simulink model "cascaded_filter"  (Simulink 6.0)
settings: Solver=ode45  StartTime=0.0  StopTime=10.0  RelTol=1e-3
model workspace (MAT data in the model file):
  L = [4.47e-09 1.86e-06 8.93e-09]
  C = [1.007e-09 2.4e-12 5.04e-10]
undefined symbols (not defined in the file or in its folder): Fs, rfckt
libraries: rfports1 x6, rfblackbox1 x4, dspsnks4 x3, rftxlines1 x2, rfladderfilters1 x1, dspsrcs4 x1
settings Model: Creator=ashivapr  LastModifiedBy=rzeng  ProdHWDeviceType=Specified  UpdateModelReferenceTargets=IfOutOfDate
settings DataIOCC: SaveOutput=off  SaveTime=off  SignalLoggingName=logsOut
settings DebuggingCC: CheckExecutionContextPreStartOutputMsg=on  CheckExecutionContextRuntimeOutputMsg=on  SolverPrmCheckMsg=none
settings HardwareCC: ProdHWDeviceType=Specified
settings ModelReferenceCC: UpdateModelReferenceTargets=IfOutOfDate
settings GRTTargetCC: UtilityFuncGeneration=Automatic  LifeSpan=inf
settings SFSimCC: SFSimApplyToAllLibs=on  SFSimBuildMode=Incremental

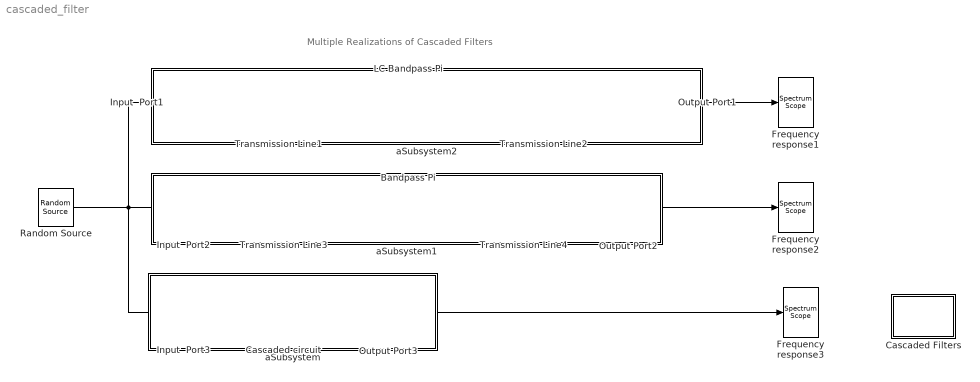
== system cascaded_filter ==
  note: Multiple Realizations of Cascaded Filters
  Bandpass Pi : rfblackbox1/General  Circuit Element  PhysicalDomain=rfsystemsdomain  SubClassName=general-circuit-element  LeftPortType=p1  RightPortType=p1  LConnTagsString=__newl0  RConnTagsString=__newr0  Ckt=rfckt.lcbandpasspi('L', L ,'C',C)  DisplayData=off  PlotFreq=Derived from Input Port parameters  PlotFreqNoSim=User specified  Freq=[70e6:1.0e5:80e6]  AllPlotType=X-Y plane  NetworkData=S21  SmithData=S11  PolarData=S11  ComplexFormat=Magnitude (decibels)  DBFormat=Magnitude (decibels)  NoneFormat=None
  Cascaded Filters : Subsystem  EnableExecutionContextPropagation=on
      mask Display: disp('Info')
  Cascaded circuit : rfblackbox1/General  Circuit Element  PhysicalDomain=rfsystemsdomain  SubClassName=general-circuit-element  LeftPortType=p1  RightPortType=p1  LConnTagsString=__newl0  RConnTagsString=__newr0  Ckt=rfckt.cascade('Ckts',{rfckt.txline,rfckt.lcbandpasspi('L', L, 'C',C), rfckt.txline})  DisplayData=off  PlotFreq=Derived from Input Port parameters  PlotFreqNoSim=User specified  Freq=[70e6:1.0e5:80e6]  AllPlotType=X-Y plane  NetworkData=S21  SmithData=S11  PolarData=S11  ComplexFormat=Magnitude (decibels)  DBFormat=Magnitude (decibels)  NoneFormat=None
  Frequency response1 : dspsnks4/Spectrum Scope  ScopeProperties=off  Domain=Frequency  HorizSpan=1  UseBuffer=off  BufferSize=128  Overlap=64  inpFftLenInherit=off  FFTlength=1024  numAvg=20  DisplayProperties=off  AxisGrid=on  Memory=off  FrameNumber=off  AxisLegend=off  AxisZoom=off  OpenScopeAtSimStart=on  OpenScopeImmediately=off  FigPos=[39 353 295 178]  AxisProperties=off  XUnits=Hertz  XRange=[-Fs/2...Fs/2]  InheritXIncr=on  XIncr=1.0  XLabel=Samples  YUnits=dB  YLabel=Magnitude, dB  LineProperties=on  LineColors=[0 0 1]
      settings: YMin=-21.8531881151715  YMax=-0.111894463142355
  Frequency response2 : dspsnks4/Spectrum Scope  ScopeProperties=off  Domain=Frequency  HorizSpan=1  UseBuffer=off  BufferSize=128  Overlap=64  inpFftLenInherit=off  FFTlength=1024  numAvg=20  DisplayProperties=off  AxisGrid=on  Memory=off  FrameNumber=off  AxisLegend=off  AxisZoom=off  OpenScopeAtSimStart=on  OpenScopeImmediately=off  FigPos=[342 353 294 178]  AxisProperties=off  XUnits=Hertz  XRange=[-Fs/2...Fs/2]  InheritXIncr=on  XIncr=1.0  XLabel=Samples  YUnits=dB  YLabel=Magnitude, dB  LineProperties=on  LineColors=[1 0 0]
      settings: YMin=-21.8644242577982  YMax=-0.721656811847852
  Frequency response3 : dspsnks4/Spectrum Scope  ScopeProperties=off  Domain=Frequency  HorizSpan=1  UseBuffer=off  BufferSize=128  Overlap=64  inpFftLenInherit=off  FFTlength=1024  numAvg=20  DisplayProperties=off  AxisGrid=on  Memory=off  FrameNumber=off  AxisLegend=off  AxisZoom=off  OpenScopeAtSimStart=on  OpenScopeImmediately=off  FigPos=[644 354 297 179]  AxisProperties=off  XUnits=Hertz  XRange=[-Fs/2...Fs/2]  InheritXIncr=on  XIncr=1.0  XLabel=Samples  YUnits=dB  YLabel=Magnitude, dB  LineProperties=on  LineColors=[0 0 0]
      settings: YMin=-21.7603958691771  YMax=-0.180062979467108
  Input  Port1 : rfports1/Input Port  Description=source block  MaxLength=128  Fc=75e6  Ts=1e-7  Zs=50  NoiseFlag=off  seed=67987  GoToTag=AAEGBHDRJLOGNSMOUDGJWHR
  Input  Port2 : rfports1/Input Port  Description=source block  MaxLength=128  Fc=75e6  Ts=1e-7  Zs=50  NoiseFlag=off  seed=67987  GoToTag=BBAACIESKMPHOTNPVEHKXIS
  Input  Port3 : rfports1/Input Port  Description=source block  MaxLength=128  Fc=75e6  Ts=1e-7  Zs=50  NoiseFlag=off  seed=67987  GoToTag=ACBBDJFALNQIAUOQWFILYJT
  LC Bandpass Pi : rfladderfilters1/LC Bandpass Pi  PhysicalDomain=rfsystemsdomain  SubClassName=lcbandpasspi  LeftPortType=p1  RightPortType=p1  LConnTagsString=__newl0  RConnTagsString=__newr0  L=L  C=C  DisplayData=off  PlotFreq=Derived from Input Port parameters  PlotFreqNoSim=User specified  Freq=[70e6:1.0e5:80e6]  AllPlotType=X-Y plane  NetworkData=S21  SmithData=S11  PolarData=S11  ComplexFormat=Magnitude (decibels)  DBFormat=Magnitude (decibels)  NoneFormat=None
  Output Port1 : rfports1/Output Port  Zl=100  num_Models=1  GoToTag=AAEGBHDRJLOGNSMOUDGJWHR  DisplayData=off  PlotFreq=Derived from Input Port parameters  Freq=1e9:1e8:3e9  AllPlotType=Composite data  NoBudgetPlot=Composite data  NetworkData=S11  SmithData=S11  PolarData=S11  ComplexFormat=Magnitude (decibels)  DBFormat=Magnitude (decibels)  DBMFormat=dBm  NoneFormat=None
  Output Port2 : rfports1/Output Port  Zl=100  num_Models=1  GoToTag=BBAACIESKMPHOTNPVEHKXIS  DisplayData=off  PlotFreq=Derived from Input Port parameters  Freq=1e9:1e8:3e9  AllPlotType=Composite data  NoBudgetPlot=Composite data  NetworkData=S11  SmithData=S11  PolarData=S11  ComplexFormat=Magnitude (decibels)  DBFormat=Magnitude (decibels)  DBMFormat=dBm  NoneFormat=None
  Output Port3 : rfports1/Output Port  Zl=100  num_Models=1  GoToTag=ACBBDJFALNQIAUOQWFILYJT  DisplayData=off  PlotFreq=Derived from Input Port parameters  Freq=1e9:1e8:3e9  AllPlotType=Composite data  NoBudgetPlot=Composite data  NetworkData=S11  SmithData=S11  PolarData=S11  ComplexFormat=Magnitude (decibels)  DBFormat=Magnitude (decibels)  DBMFormat=dBm  NoneFormat=None
  Random Source : dspsrcs4/Random Source  SrcType=Gaussian  NormMethod=Ziggurat  CltLength=12  Min=0  Max=1  Mean=0  Var=1  RepMode=Not repeatable  Seed=1  Inherit=off  SampMode=Discrete  SampTime=1e-7  SampFrame=256  DataType=Double  OutComplex=Complex
  Transmission Line1 : rftxlines1/Transmission Line  PhysicalDomain=rfsystemsdomain  SubClassName=txline  LeftPortType=p1  RightPortType=p1  LConnTagsString=__newl0  RConnTagsString=__newr0  Z0=50  PV=299792458  Loss=0  LineLength=0.01  StubMode=Not a stub  Termination=Open  DisplayData=off  PlotFreq=Derived from Input Port parameters  PlotFreqNoSim=User specified  Freq=[70e6:1.0e5:80e6]  AllPlotType=X-Y plane  NetworkData=S21  SmithData=S11  PolarData=S11  ComplexFormat=Magnitude (decibels)  DBFormat=Magnitude (decibels)  NoneFormat=None
  Transmission Line2 : rftxlines1/Transmission Line  PhysicalDomain=rfsystemsdomain  SubClassName=txline  LeftPortType=p1  RightPortType=p1  LConnTagsString=__newl0  RConnTagsString=__newr0  Z0=50  PV=299792458  Loss=0  LineLength=0.01  StubMode=Not a stub  Termination=Open  DisplayData=off  PlotFreq=Derived from Input Port parameters  PlotFreqNoSim=User specified  Freq=[70e6:1.0e5:80e6]  AllPlotType=X-Y plane  NetworkData=S21  SmithData=S11  PolarData=S11  ComplexFormat=Magnitude (decibels)  DBFormat=Magnitude (decibels)  NoneFormat=None
  Transmission Line3 : rfblackbox1/General  Circuit Element  PhysicalDomain=rfsystemsdomain  SubClassName=general-circuit-element  LeftPortType=p1  RightPortType=p1  LConnTagsString=__newl0  RConnTagsString=__newr0  Ckt=rfckt.txline  DisplayData=off  PlotFreq=Derived from Input Port parameters  PlotFreqNoSim=User specified  Freq=[70e6:1.0e5:80e6]  AllPlotType=X-Y plane  NetworkData=S21  SmithData=S11  PolarData=S11  ComplexFormat=Magnitude (decibels)  DBFormat=Magnitude (decibels)  NoneFormat=None
  Transmission Line4 : rfblackbox1/General  Circuit Element  PhysicalDomain=rfsystemsdomain  SubClassName=general-circuit-element  LeftPortType=p1  RightPortType=p1  LConnTagsString=__newl0  RConnTagsString=__newr0  Ckt=rfckt.txline  DisplayData=off  PlotFreq=Derived from Input Port parameters  PlotFreqNoSim=User specified  Freq=[70e6:1.0e5:80e6]  AllPlotType=X-Y plane  NetworkData=S21  SmithData=S11  PolarData=S11  ComplexFormat=Magnitude (decibels)  DBFormat=Magnitude (decibels)  NoneFormat=None
  aSubsystem : Subsystem  EnableExecutionContextPropagation=on
      mask Display: disp('')
  aSubsystem1 : Subsystem  EnableExecutionContextPropagation=on
      mask Display: disp('')
  aSubsystem2 : Subsystem  EnableExecutionContextPropagation=on
      mask Display: disp('')
  wires:
  Random Source/1 -> Input  Port1/1, Input  Port2/1, Input  Port3/1
  Output Port3/1 -> Frequency response3/1
  Output Port2/1 -> Frequency response2/1
  Output Port1/1 -> Frequency response1/1
  connections:
  Input  Port2/RConn1 -- Transmission Line3/LConn1
  Transmission Line3/RConn1 -- Bandpass Pi/LConn1
  Bandpass Pi/RConn1 -- Transmission Line4/LConn1
  Transmission Line4/RConn1 -- Output Port2/LConn1
  Transmission Line1/LConn1 -- Input  Port1/RConn1
  Transmission Line1/RConn1 -- LC Bandpass Pi/LConn1
  LC Bandpass Pi/RConn1 -- Transmission Line2/LConn1
  Transmission Line2/RConn1 -- Output Port1/LConn1
  Input  Port3/RConn1 -- Cascaded circuit/LConn1
  Cascaded circuit/RConn1 -- Output Port3/LConn1

== system cascaded_filter/Cascaded Filters ==
  note: Multiple Realizations of Cascaded Filters
  note: This model illustrates three different ways to create a
      | cascade of three filters - the transmission line, bandpass
      | filter and another transmission line.
  note: The first method uses transmission line blocks
      | from the Transmission Lines sublibrary and bandpass
      | filter block from the Ladder Filters sublibrary.
  note: The second method creates transmission line and bandpass
      | filter objects using the General Circuit Element block from
      | Black Box Elements sublibrary and the RF Toolbox objects.
  note: The third method creates a cascade object using the General
      | Circuit Element block and RF Toolbox objects

== system cascaded_filter/aSubsystem ==

== system cascaded_filter/aSubsystem1 ==

== system cascaded_filter/aSubsystem2 ==
